simulink model "uavSafeLanding"  (R2023b)
settings: Solver=VariableStepAuto  StartTime=0.0  StopTime=inf  RelTol=1e-3
values from neighbouring files (symbols this model uses):
  DroneMass = 0.1    [controllerData.sldd]
  Dx = 1.5    [controllerData.sldd]
  Dy = 1.5    [controllerData.sldd]
  Dz = 2.5    [controllerData.sldd]
  Gravity = 9.81    [controllerData.sldd]
  Ix = 0.0    [controllerData.sldd]
  Iy = 0.0    [controllerData.sldd]
  Iz = 0.0    [controllerData.sldd]
  Nx = 10.0    [controllerData.sldd]
  Ny = 10.0    [controllerData.sldd]
  Nz = 14.4947065605712    [controllerData.sldd]
  Px = 6.0    [controllerData.sldd]
  Py = 6.0    [controllerData.sldd]
  Pz = 6.5    [controllerData.sldd]
undefined symbols (not defined in the file or in its folder): mission, rigidtform3d
libraries: slpidlib x6, uavalgslib x3, robotcorelib x2, simulink x1, sim3dphyssensorlib x1, sim3dlib x1, uavsim3dlib x1, uavutilslib x1
settings Model: DataDictionary=controllerData.sldd  Creator=The MathWorks, Inc.  LastModifiedBy=The MathWorks, Inc.
settings DebuggingCC: ParameterPrecisionLossMsg=none

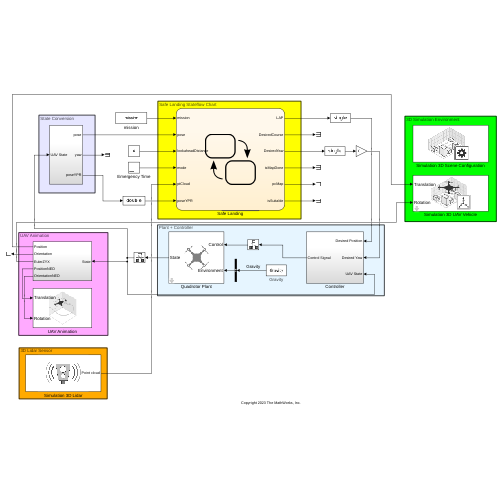
[thumbnail: Simulink's stored preview of the top-level diagram]
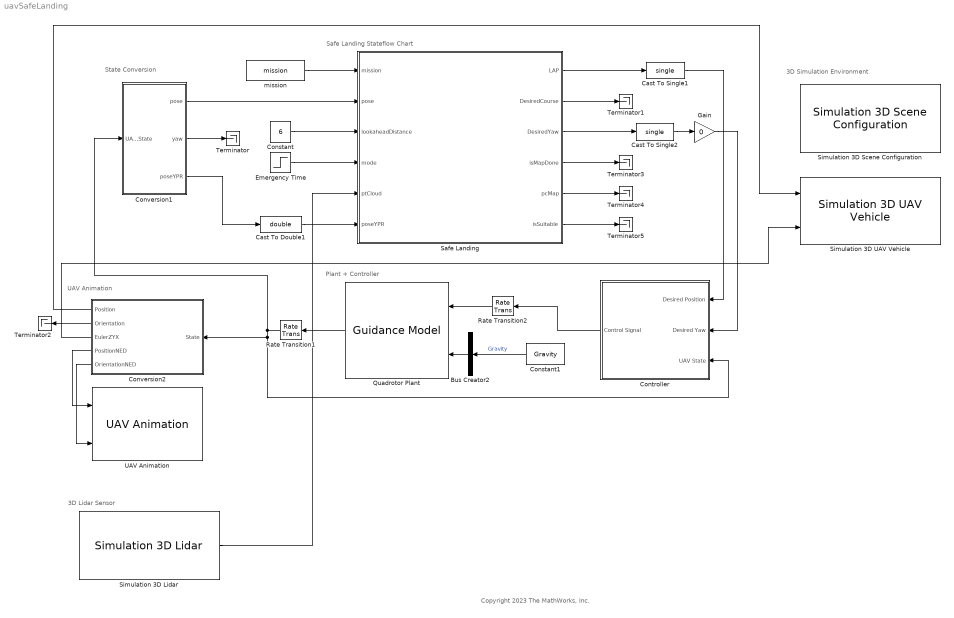
== system uavSafeLanding ==
  note: UAV Animation
  note: 3D Lidar Sensor
  note: Plant + Controller
  note: State Conversion
  note: 3D Simulation Environment
  note: Safe Landing Stateflow Chart
  note: Copyright 2023 The MathWorks, Inc.
  Bus Creator2 : BusCreator  Inputs=1  OutDataTypeStr=Bus: uavGuidanceEnvironmentBus  NonVirtualBus=on
  Cast To Double1 : DataTypeConversion  OutDataTypeStr=double  SaturateOnIntegerOverflow=off  RndMeth=Floor
  Cast To Single1 : DataTypeConversion  OutDataTypeStr=single  SaturateOnIntegerOverflow=off  RndMeth=Floor
  Cast To Single2 : DataTypeConversion  OutDataTypeStr=single  SaturateOnIntegerOverflow=off  RndMeth=Floor
  Constant : Constant  Value=6
  Constant1 : Constant  Value=Gravity  OutDataTypeStr=single
      settings: AttributesFormatString=%<Value>
  Controller : Subsystem
  Conversion1 : Subsystem
  Conversion2 : Subsystem
  Emergency Time : Step  Time=Time  Before=1  After=2  SampleTime=0  mask{Time=10}
      mask prompts: Time "Emergency time (s):"
      mask TypeOptions Time: Time
  Gain : Gain  Gain=0
  Quadrotor Plant : uavalgslib/Guidance Model  ModelType=MultirotorGuidance  SpecifiedDataType=single  SimulateUsing=Code generation  InitialWorldPositionMultirotor=[mission(1,1);mission(1,2);mission(1,3)]  InitialWorldVelocityMultirotor=[0; 0; 0]  InitialEulerZYXMultirotor=|  InitialBodyAngularRateRPYMultirotor=[0; 0; 0]  InitialThrustMultirotor=0  InitialNorthFixedWing=0  InitialEastFixedWing=0  InitialHeightFixedWing=0  InitialAirSpeedFixedWing=0  InitialHeadingAngleFixedWing=0  InitialFlightPathAngleFixedWing=0  InitialRollAngleFixedWing=0  InitialRollAngleRateFixedWing=0  PDRollMultirotor=[3402.97,116.67]  PDPitchMultirotor=[3402.97, 116.67]  PYawRateMultirotor=1950  PThrustMultirotor=3900  MassMultirotor=0.1  PHeightFixedWing=3.9  PHeadingAngleFixedWing=3.9  PFlightPathAngleFixedWing=39  PDRollFixedWing=[3402.97, 116.67]  PAirSpeedFixedWing=1  FlightPathAngleLimitsFixedWing=[-pi/2, pi/2]  StateBusName='uavGuidanceStateBus'  ControlBusName='uavGuidanceControlBus'  EnvironmentBusName='uavGuidanceEnvironmentBus'  DataType=single
      | [ 0
      | ;0;0]
  Rate Transition1 : RateTransition  OutPortSampleTime=UAVSampleTime
  Rate Transition2 : RateTransition  OutPortSampleTime=UAVSampleTime
  Safe Landing : Stateflow chart  TreatAsAtomicUnit=on  SystemSampleTime=0.1
  Simulation 3D Lidar : sim3dphyssensorlib/Simulation 3D Lidar  Priority=1  sensorTag=Sim3dSensor1  sensorId=1  sensorName=Sim3dSensor1  vehTagList={'Scene Origin';'SimulinkVehicle1'}  vehTag=SimulinkVehicle1  mountLoc=Origin  offsetFlag=on  tmountOffset=[0, 0, -1]  rmountOffset=[0, 90, 0]  DetectionRange=100  RangeResolution=0.03  VerticalFOV=30  VerticalResolution=2  HorizontalFOV=360  HorizontalResolution=0.2  DistanceOutportEnabled=off  ReflectivityOutportEnabled=off  SemanticOutportEnabled=off  TransformOutportEnabled=off  SampleTime=0.1  mountPoint=[0 0 -1]  mountOrientation=[0 -90 0]  aMode=4  ID=1
      settings: LibrarySourceBlock=uavsim3dlib/Simulation 3D Lidar
  Simulation 3D Scene Configuration : sim3dlib/Simulation 3D Scene Configuration  Priority=0  ProjectFormat=Default Scenes  SceneDesc=US city block  ProjectName=/mathworks/devel/bat/Bdoc23b/build/matlab/toolbox/shared/sim3d_projects/automotive_project_linux/UE/LinuxNoEditor/AutoVrtlEnv.sh  ScenePath=/Game/Maps/USCityBlock  EnableOpenDRIVE=off  vehTagList={'Custom';'Scene Origin';'SimulinkVehicle1'}  vehTag=SimulinkVehicle1  FreeCameraInitialTranslation=[0, 0, 0]  FreeCameraDefaultInitialTranslation=[-6, 0, 2]  FreeCameraInitialRotation=[0, 0, 0]  FreeCameraDefaultInitialRotation=[0, -15, 0]  OpVisEn=off  Ts=0.1  EnableWindow=on  EnableRemoteAccess=off  EnableWeather=off  SunAltitude=-57.600  SunAzimuth=90  clouds=67.0  wind=1  fog=98.0  rain=88.0  EnableGeospatial=off  OriginHeight=200  OriginLatitude=40.744652  OriginLongitude=-73.988864  MapStyle=Aerial  AdditionalAssetIDs=[]  UseAdvancedSunSky=off  SolarTime=11  TimeZone=-5  Day=21  Month=9  Year=2022  UseDaylightSavingTime=on  DSTStartDay=10  DSTStartMonth=3  DSTEndDay=3  DSTEndMonth=11  DSTSwitchHour=2  sensorTag=MainCamera1  sensorId=1  sensorName=MainCamera1  mountLoc=Origin  offsetFlag=off  tmountOffset=[0, 0, 0]  rmountOffset=[0, 0, 0]  HorizontalResolution=1280  VerticalResolution=720  HorizontalFOV=60  mountPoint=[0 0 0]  mountOrientation=[0 0 0]  aMode=4  ID=1  GeoTrigger=Inactive
      settings: LibrarySourceBlock=uavsim3dlib/Simulation 3D Scene Configuration
  Simulation 3D UAV Vehicle : uavsim3dlib/Simulation 3D UAV Vehicle  Priority=-1  Mesh=Quadrotor  MeshPath=/MathWorksUAVContent/UAVs/HexaRotorUAV/HexaRotor.HexaRotor  Color=Yellow  ActorName=SimulinkVehicle1  UseGlobalFrame=off  InitialTranslation=[mission(1,1) mission(1,2) mission(1,3)]  InitialRotation=[0 0 0]  InitialTranslationGlobal=[0 0 0]  InitialGeoOrigin=[0 0 0]  InitialRotationGlobal=[0 0 0]  SampleTime=-1  ActorType=SimulinkVehicle  ID=1  aMode=4  ActorTag=SimulinkVehicle1
  Terminator{,1..5} (6 alike) : Terminator
  UAV Animation : uavutilslib/UAV Animation  UAVType=Multirotor  UAVSize=1  InertialZDirection=Down  SampleTime=0.2
  mission : Constant  Value=mission
  wires:
  Emergency Time/1 -> Safe Landing/4(mode)
  Conversion1/2(yaw) -> Terminator/1
  Constant1/1 -> Bus Creator2/1  "Gravity"
  Cast To Single2/1 -> Gain/1
  Rate Transition2/1 -> Quadrotor Plant/1
  Conversion2/1(Position) -> Simulation 3D UAV Vehicle/1
  Safe Landing/3(DesiredYaw) -> Cast To Single2/1
  Cast To Single1/1 -> Controller/1(Desired Position)
  Conversion1/1(pose) -> Safe Landing/2(pose)
  Safe Landing/2(DesiredCourse) -> Terminator1/1
  Bus Creator2/1 -> Quadrotor Plant/2
  Rate Transition1/1 -> Controller/3(UAV State), Conversion2/1(State), Conversion1/1(UAV State)
  Gain/1 -> Controller/2(Desired Yaw)
  Constant/1 -> Safe Landing/3(lookaheadDistance)
  mission/1 -> Safe Landing/1(mission)
  Quadrotor Plant/1 -> Rate Transition1/1
  Controller/1(Control Signal) -> Rate Transition2/1
  Safe Landing/1(LAP) -> Cast To Single1/1
  Conversion1/3(poseYPR) -> Cast To Double1/1
  Cast To Double1/1 -> Safe Landing/6(poseYPR)
  Simulation 3D Lidar/1 -> Safe Landing/5(ptCloud)
  Conversion2/3(EulerZYX) -> Simulation 3D UAV Vehicle/2
  Conversion2/2(Orientation) -> Terminator2/1
  Safe Landing/4(isMapDone) -> Terminator3/1
  Safe Landing/5(pcMap) -> Terminator4/1
  Safe Landing/6(isSuitable) -> Terminator5/1
  Conversion2/4(PositionNED) -> UAV Animation/1
  Conversion2/5(OrientationNED) -> UAV Animation/2

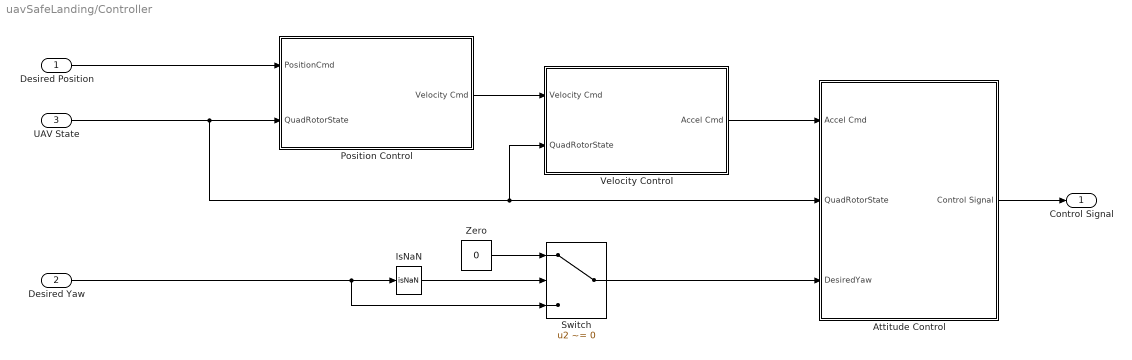
== system uavSafeLanding/Controller ==
  Desired Position : Inport
  Desired Yaw : Inport  Port=2
  UAV State : Inport  Port=3
  Attitude Control : Subsystem
  IsNaN : RelationalOperator  Operator=isNaN  OutDataTypeStr=boolean  RndMeth=Simplest  InputSameDT=off
  Position Control : Subsystem
  Switch : Switch  Criteria=u2 ~= 0  SaturateOnIntegerOverflow=off  InputSameDT=off
  Velocity Control : Subsystem
  Zero : Constant  Value=0  OutDataTypeStr=Inherit: Inherit via back propagation
  Control Signal : Outport
  wires:
  Desired Position/1 -> Position Control/1(PositionCmd)
  Velocity Control/1(Accel Cmd) -> Attitude Control/1(Accel Cmd)
  Attitude Control/1(Control Signal) -> Control Signal/1
  UAV State/1 -> Position Control/2(QuadRotorState), Velocity Control/2(QuadRotorState), Attitude Control/2(QuadRotorState)
  Position Control/1(Velocity Cmd) -> Velocity Control/1(Velocity Cmd)
  Zero/1 -> Switch/1
  IsNaN/1 -> Switch/2
  Desired Yaw/1 -> Switch/3, IsNaN/1
  Switch/1 -> Attitude Control/3(DesiredYaw)

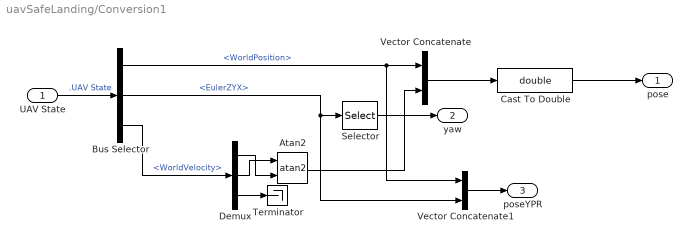
== system uavSafeLanding/Conversion1 ==
  UAV State : Inport
  Atan2 : Trigonometry  Operator=atan2
  Bus Selector : BusSelector  OutputSignals=WorldPosition,EulerZYX,WorldVelocity
  Cast To Double : DataTypeConversion  OutDataTypeStr=double  SaturateOnIntegerOverflow=off  RndMeth=Floor
  Demux : Demux  Outputs=3
  Selector : Selector  InputPortWidth=3  IndexOptions=Index vector (dialog)  Indices=[1]  OutputSizes=1
  Terminator : Terminator
  Vector Concatenate : Concatenate
  Vector Concatenate1 : Concatenate
  pose : Outport
  yaw : Outport  Port=2
  poseYPR : Outport  Port=3
  wires:
  Bus Selector/2 -> Vector Concatenate1/2, Selector/1  "<EulerZYX>"
  Bus Selector/1 -> Vector Concatenate1/1, Vector Concatenate/1  "<WorldPosition>"
  UAV State/1 -> Bus Selector/1  ".UAV State"
  Vector Concatenate/1 -> Cast To Double/1
  Bus Selector/3 -> Demux/1  "<WorldVelocity>"
  Demux/3 -> Terminator/1
  Atan2/1 -> Vector Concatenate/2
  Selector/1 -> yaw/1
  Demux/2 -> Atan2/1
  Demux/1 -> Atan2/2
  Vector Concatenate1/1 -> poseYPR/1
  Cast To Double/1 -> pose/1

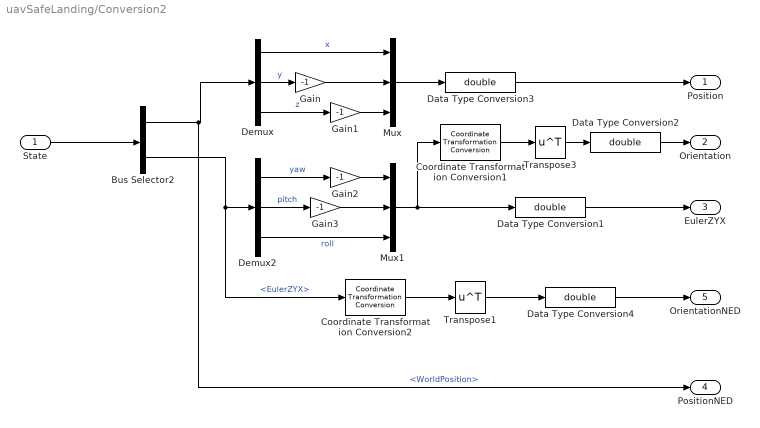
== system uavSafeLanding/Conversion2 ==
  State : Inport
  Bus Selector2 : BusSelector  OutputSignals=WorldPosition,EulerZYX
  Coordinate Transformation Conversion1 : robotcorelib/Coordinate Transformation Conversion  InputRepresentation=Euler Angles  InputEulerSequence=ZYX  ShowTrVecInputPort=on  OutputRepresentation=Quaternion  OutputEulerSequence=ZYX  ShowTrVecOutputPort=on  SimulateUsing=Code generation
  Coordinate Transformation Conversion2 : robotcorelib/Coordinate Transformation Conversion  InputRepresentation=Euler Angles  InputEulerSequence=ZYX  ShowTrVecInputPort=on  OutputRepresentation=Quaternion  OutputEulerSequence=ZYX  ShowTrVecOutputPort=on  SimulateUsing=Code generation
  Data Type Conversion{1..4} (4 alike) : DataTypeConversion  OutDataTypeStr=double  SaturateOnIntegerOverflow=off  RndMeth=Floor
  Demux : Demux  Outputs=3
  Demux2 : Demux  Outputs=3
  Gain{,1..3} (4 alike) : Gain  Gain=-1
  Mux : Mux  Inputs=3
  Mux1 : Mux  Inputs=3
  Transpose1 : Math  Operator=transpose
  Transpose3 : Math  Operator=transpose
  Position : Outport
  Orientation : Outport  Port=2
  EulerZYX : Outport  Port=3
  PositionNED : Outport  Port=4
  OrientationNED : Outport  Port=5
  wires:
  Bus Selector2/1 -> PositionNED/1, Demux/1  "<WorldPosition>"
  Gain3/1 -> Mux1/2
  Demux2/3 -> Mux1/3  "roll"
  State/1 -> Bus Selector2/1
  Demux/2 -> Gain/1  "y"
  Gain1/1 -> Mux/3
  Gain/1 -> Mux/2
  Demux/1 -> Mux/1  "x"
  Gain2/1 -> Mux1/1
  Demux2/1 -> Gain2/1  "yaw"
  Demux/3 -> Gain1/1  "z"
  Demux2/2 -> Gain3/1  "pitch"
  Mux/1 -> Data Type Conversion3/1
  Coordinate Transformation Conversion1/1 -> Transpose3/1
  Bus Selector2/2 -> Coordinate Transformation Conversion2/1, Demux2/1  "<EulerZYX>"
  Transpose3/1 -> Data Type Conversion2/1
  Mux1/1 -> Coordinate Transformation Conversion1/1, Data Type Conversion1/1
  Data Type Conversion3/1 -> Position/1
  Data Type Conversion2/1 -> Orientation/1
  Data Type Conversion1/1 -> EulerZYX/1
  Coordinate Transformation Conversion2/1 -> Transpose1/1
  Transpose1/1 -> Data Type Conversion4/1
  Data Type Conversion4/1 -> OrientationNED/1

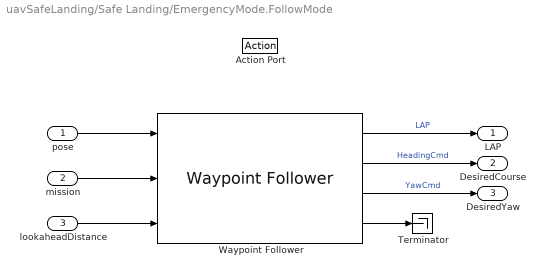
== system uavSafeLanding/Safe Landing/EmergencyMode.FollowMode ==
  pose : Inport
  mission : Inport  Port=2
  lookaheadDistance : Inport  Port=3
  Action Port : ActionPort
      settings: CopyFcn=Stateflow.SLINSF.SimulinkMan.removeBlockPreDeleteFcn  PreDeleteFcn=Stateflow.SLINSF.SimulinkMan.unsafePredeleteFcn
  Terminator : Terminator
  Waypoint Follower : uavalgslib/Waypoint Follower  UAVType=multirotor  StartFrom=closest  TransitionRadiusSource=internal  TransitionRadius=5  MinLookaheadDistance=0.1  YawInput=off  ShowCrossTrackErrorOutput=off  ShowStatusOutput=off  SimulateUsing=Interpreted execution
  LAP : Outport
  DesiredCourse : Outport  Port=2
  DesiredYaw : Outport  Port=3
  wires:
  mission/1 -> Waypoint Follower/2
  lookaheadDistance/1 -> Waypoint Follower/3
  Waypoint Follower/1 -> LAP/1  "LAP"
  pose/1 -> Waypoint Follower/1
  Waypoint Follower/4 -> Terminator/1
  Waypoint Follower/3 -> DesiredYaw/1  "YawCmd"
  Waypoint Follower/2 -> DesiredCourse/1  "HeadingCmd"

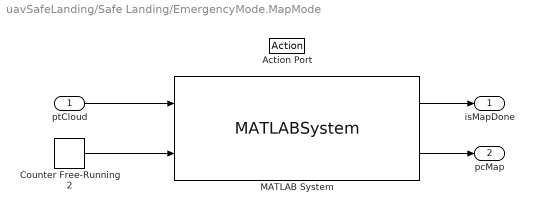
== system uavSafeLanding/Safe Landing/EmergencyMode.MapMode ==
  ptCloud : Inport
  Action Port : ActionPort
      settings: CopyFcn=Stateflow.SLINSF.SimulinkMan.removeBlockPreDeleteFcn  PreDeleteFcn=Stateflow.SLINSF.SimulinkMan.unsafePredeleteFcn
  Counter Free-Running2 : simulink/Sources/Counter Free-Running  NumBits=16  tsamp=-1
  MATLAB System : MATLABSystem  System=exampleHelperMapBuilder  mapGridSize=0.2  downsamplePercent=0.1  quadCopterROI=[ -2, 2, -2, 2, -2, 2 ]  sensorPoseWRTUAV=rigidtform3d( [ 90, 90, 0 ], [ 0, 0, 0 ] )  SimulateUsing=Interpreted execution
      mask Type: exampleHelperMapBuilder
      mask Display:
      | disp('exampleHelperMapBuilder');
      | port_label('input',1,'ptcloud');
      | port_label('input',2,'count');
      | port_label('output',1,'isMapDone');
      | port_label('output',2,'pcMap');
  isMapDone : Outport  OutDataTypeStr=boolean  PortDimensions=[1 1]
      settings: VarSizeSig=Yes
  pcMap : Outport  Port=2  OutDataTypeStr=double  PortDimensions=[600000 3]
  wires:
  ptCloud/1 -> MATLAB System/1
  Counter Free-Running2/1 -> MATLAB System/2
  MATLAB System/1 -> isMapDone/1
  MATLAB System/2 -> pcMap/1

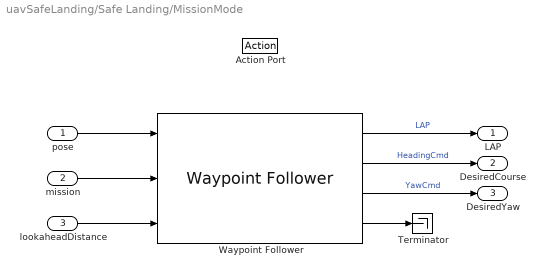
== system uavSafeLanding/Safe Landing/MissionMode ==
  pose : Inport
  mission : Inport  Port=2
  lookaheadDistance : Inport  Port=3
  Action Port : ActionPort
      settings: CopyFcn=Stateflow.SLINSF.SimulinkMan.removeBlockPreDeleteFcn  PreDeleteFcn=Stateflow.SLINSF.SimulinkMan.unsafePredeleteFcn
  Terminator : Terminator
  Waypoint Follower : uavalgslib/Waypoint Follower  UAVType=multirotor  StartFrom=first  TransitionRadiusSource=internal  TransitionRadius=5  MinLookaheadDistance=0.1  YawInput=off  ShowCrossTrackErrorOutput=off  ShowStatusOutput=off  SimulateUsing=Interpreted execution
  LAP : Outport
  DesiredCourse : Outport  Port=2
  DesiredYaw : Outport  Port=3
  wires:
  mission/1 -> Waypoint Follower/2
  lookaheadDistance/1 -> Waypoint Follower/3
  Waypoint Follower/1 -> LAP/1  "LAP"
  pose/1 -> Waypoint Follower/1
  Waypoint Follower/4 -> Terminator/1
  Waypoint Follower/3 -> DesiredYaw/1  "YawCmd"
  Waypoint Follower/2 -> DesiredCourse/1  "HeadingCmd"

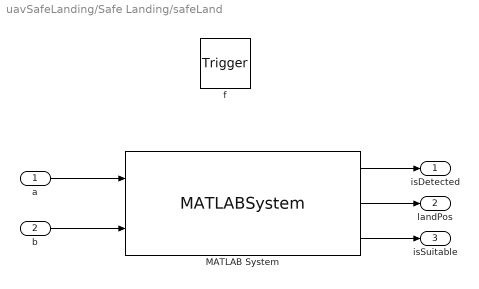
== system uavSafeLanding/Safe Landing/safeLand ==
  a : Inport  OutDataTypeStr=double  PortDimensions=[600000 3]
  b : Inport  Port=2  OutDataTypeStr=double  PortDimensions=[3 1]
  f : TriggerPort  TriggerType=function-call  VariantControl=(inherit)
      settings: CopyFcn=Stateflow.SLINSF.SimulinkMan.removeBlockPreDeleteFcn  PreDeleteFcn=Stateflow.SLINSF.SimulinkMan.unsafePredeleteFcn
  MATLAB System : MATLABSystem  System=exampleHelperSafeLanding  innerBlockSize=[ 20, 20 ]  radius=5  gridSize=3  minPoints=10  verticalVarianceThreshold=0.5  slopeThreshold=6  residualThreshold=10  reliefThreshold=3  weight=[ 1, 1, 1, 1 ]  qualityThreshold=1  pcDownsamplePercent=0.1  SimulateUsing=Interpreted execution
      mask Type: exampleHelperSafeLanding
      mask Display:
      | disp('exampleHelperSafeLanding');
      | port_label('input',1,'ptCloudMap');
      | port_label('input',2,'uavStartPosition');
      | port_label('output',1,'isDetected');
      | port_label('output',2,'bestLandingZone');
      | port_label('output',3,'isSuitable');
  isDetected : Outport
  landPos : Outport  Port=2
  isSuitable : Outport  Port=3
  wires:
  a/1 -> MATLAB System/1
  b/1 -> MATLAB System/2
  MATLAB System/1 -> isDetected/1
  MATLAB System/2 -> landPos/1
  MATLAB System/3 -> isSuitable/1

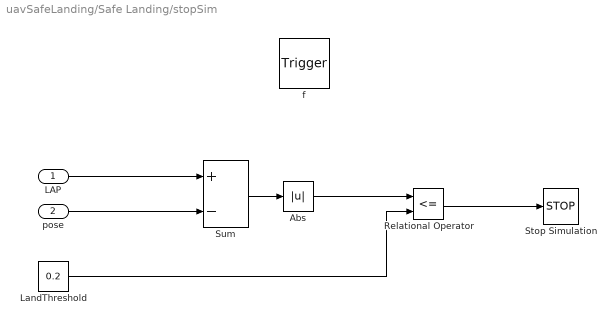
== system uavSafeLanding/Safe Landing/stopSim ==
  LAP : Inport  OutDataTypeStr=double  PortDimensions=1
  pose : Inport  Port=2  OutDataTypeStr=double  PortDimensions=1
  f : TriggerPort  TriggerType=function-call  VariantControl=(inherit)
      settings: CopyFcn=Stateflow.SLINSF.SimulinkMan.removeBlockPreDeleteFcn  PreDeleteFcn=Stateflow.SLINSF.SimulinkMan.unsafePredeleteFcn
  Abs : Abs  SaturateOnIntegerOverflow=off
  LandThreshold : Constant  Value=0.2
  Relational Operator : RelationalOperator  Operator=<=  OutDataTypeStr=boolean  RndMeth=Simplest  InputSameDT=off
  Stop Simulation : Stop
  Sum : Sum  Inputs=+-
  wires:
  LandThreshold/1 -> Relational Operator/2
  Relational Operator/1 -> Stop Simulation/1
  LAP/1 -> Sum/1
  Sum/1 -> Abs/1
  Abs/1 -> Relational Operator/1
  pose/1 -> Sum/2

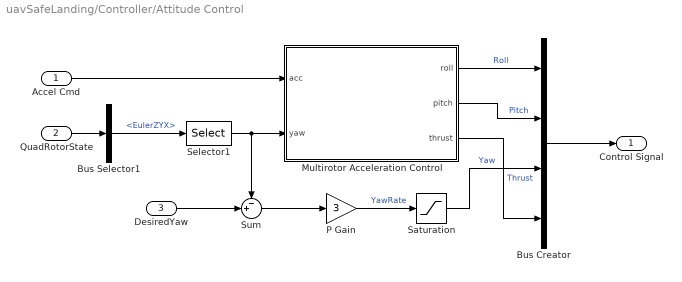
== system uavSafeLanding/Controller/Attitude Control ==
  Accel Cmd : Inport
  QuadRotorState : Inport  Port=2
  DesiredYaw : Inport  Port=3
  Bus Creator : BusCreator  Inputs=4  OutDataTypeStr=Bus: uavGuidanceControlBus  NonVirtualBus=on
      settings: InheritFromInputs=off
  Bus Selector1 : BusSelector  OutputSignals=EulerZYX
  Multirotor Acceleration Control : MATLAB Function  TreatAsAtomicUnit=on
  P Gain : Gain  Gain=3
  Saturation : Saturate
  Selector1 : Selector  InputPortWidth=3  IndexOptions=Index vector (dialog)  Indices=[1]  OutputSizes=1
  Sum : Sum  Inputs=-+|
  Control Signal : Outport
  wires:
  Selector1/1 -> Multirotor Acceleration Control/2(yaw), Sum/1
  Bus Creator/1 -> Control Signal/1
  Sum/1 -> P Gain/1
  Multirotor Acceleration Control/1(roll) -> Bus Creator/1  "Roll"
  Multirotor Acceleration Control/2(pitch) -> Bus Creator/2  "Pitch"
  Multirotor Acceleration Control/3(thrust) -> Bus Creator/4  "Thrust"
  P Gain/1 -> Saturation/1  "YawRate"
  Accel Cmd/1 -> Multirotor Acceleration Control/1(acc)
  QuadRotorState/1 -> Bus Selector1/1
  Bus Selector1/1 -> Selector1/1  "<EulerZYX>"
  Saturation/1 -> Bus Creator/3  "Yaw"
  DesiredYaw/1 -> Sum/2

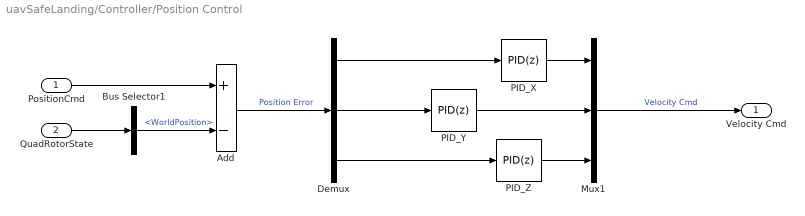
== system uavSafeLanding/Controller/Position Control ==
  PositionCmd : Inport
  QuadRotorState : Inport  Port=2
  Add : Sum  Inputs=+-
  Bus Selector1 : BusSelector  OutputSignals=WorldPosition
  Demux : Demux  Outputs=3
  Mux1 : Mux  Inputs=3
  PID_X : slpidlib/PID Controller  Controller=PID  Form=Parallel  TimeDomain=Discrete-time  UseExternalTs=off  SampleTime=-1  IntegratorMethod=Forward Euler  FilterMethod=Forward Euler  ControllerParametersSource=internal  P=Px  I=Ix  UseKiTs=off  D=Dx  N=Nx  UseFilter=on  TunerSelectOption=Transfer Function Based (PID Tuner App)  InitialConditionSource=internal  InitialConditionForIntegrator=0  InitialConditionForFilter=0  DifferentiatorICPrevScaledInput=0  ExternalReset=none  TrackingMode=off  Kt=1  LimitOutput=on  SatLimitsSource=internal  UpperSaturationLimit=3  LowerSaturationLimit=-3  LinearizeAsGain=on  AntiWindupMode=clamping  Kb=1  LimitIntegrator=off  UpperIntegratorSaturationLimit=inf  LowerIntegratorSaturationLimit=-inf  POutMin=[]  POutMax=[]  IOutMin=[]  IOutMax=[]  DOutMin=[]  DOutMax=[]  NOutMin=[]  NOutMax=[]  SumOutMin=[]  SumOutMax=[]  SaturationOutMin=[]  SaturationOutMax=[]  PParamMin=[]  PParamMax=[]  IParamMin=[]  IParamMax=[]  DParamMin=[]  DParamMax=[]  NParamMin=[]  NParamMax=[]  KbParamMin=[]  KbParamMax=[]  KtParamMin=[]  KtParamMax=[]  KbOutMin=[]  KbOutMax=[]  KtOutMin=[]  KtOutMax=[]  IntegratorOutMin=[]  IntegratorOutMax=[]  FilterOutMin=[]  FilterOutMax=[]  SumI1OutMin=SumI1OutMin  SumI1OutMax=SumI1OutMax  SumI2OutMin=[]  SumI2OutMax=[]  SumI3OutMin=[]  SumI3OutMax=[]  SumI4OutMin=[]  SumI4OutMax=[]  SumDOutMin=[]  SumDOutMax=[]  DifferentiatorOutMin=[]  DifferentiatorOutMax=[]  FilterDiffOutCoefMin=[]  FilterDiffOutCoefMax=[]  ReciprocalOutMin=[]  ReciprocalOutMax=[]  SumDenOutMin=[]  SumDenOutMax=[]  SumNumOutMin=[]  SumNumOutMax=[]  DivideOutMin=[]  DivideOutMax=[]  UdiffTsProdOutMin=[]  UdiffTsProdOutMax=[]  NTsProdOutMin=[]  NTsProdOutMax=[]  UintegralTsProdOutMin=[]  UintegralTsProdOutMax=[]  UngainTsProdOutMin=[]  UngainTsProdOutMax=[]  ClampingZeroOutDataTypeStr=Inherit: Inherit via back propagation  ClampingZeroOutMin=[]  ClampingZeroOutMax=[]  FilterDenConstantOutDataTypeStr=Inherit: Inherit via back propagation  FilterDenConstantOutMin=[]  FilterDenConstantOutMax=[]  PCopyOutDataTypeStr=Inherit: Inherit via back propagation  PCopyOutMin=[]  PCopyOutMax=[]  NCopyOutDataTypeStr=Inherit: Inherit via back propagation  NCopyOutMin=[]  NCopyOutMax=[]  IntegratorContinuousStateAttributes=''  IntegratorStateMustResolveToSignalObject=off  IntegratorRTWStateStorageClass=Auto  FilterContinuousStateAttributes=''  FilterStateMustResolveToSignalObject=off  FilterRTWStateStorageClass=Auto  ParallelPVariant=InternalParameters  IdealPVariant=Disabled  IVariant=InternalParameters  DVariant=InternalParameters  IntegratorVariant=Discrete  SatVariant=Enabled  AWVariant=DiscClampingParallel  PCopyVariant=Disabled  TRVariant=Disabled  FdbkBlocksVariant=Forward  IdealPFdbkVariant=Disabled  SatFdbkVariant=Disabled  DerivativeFilterVariant=ForwardEulerFilter  NVariant=InternalParameters  NCopyVariant=Disabled  FilterICVariant=InternalICsFilter  IntegratorICVariant=InternalICs  ExternalResetVariant=Disabled  TRSumVariant=Passthrough  SumFdbkVariant=Disabled  SumVariant=Sum_PID  TsampFilterVariant=InternalTs  TsampNgainVariant=Passthrough  TsampIntegralVariant=Disabled_SignalSpec  ExternalSaturationOutDataTypeStr=Inherit: Same as second input
      settings: AttributesFormatString=P: %<P>, I: %<I>, D:%<D>
  PID_Y : slpidlib/PID Controller  Controller=PID  Form=Parallel  TimeDomain=Discrete-time  UseExternalTs=off  SampleTime=-1  IntegratorMethod=Forward Euler  FilterMethod=Forward Euler  ControllerParametersSource=internal  P=Py  I=Iy  UseKiTs=off  D=Dy  N=Ny  UseFilter=on  TunerSelectOption=Transfer Function Based (PID Tuner App)  InitialConditionSource=internal  InitialConditionForIntegrator=0  InitialConditionForFilter=0  DifferentiatorICPrevScaledInput=0  ExternalReset=none  TrackingMode=off  Kt=1  LimitOutput=on  SatLimitsSource=internal  UpperSaturationLimit=3  LowerSaturationLimit=-3  LinearizeAsGain=on  AntiWindupMode=clamping  Kb=1  LimitIntegrator=off  UpperIntegratorSaturationLimit=inf  LowerIntegratorSaturationLimit=-inf  POutMin=[]  POutMax=[]  IOutMin=[]  IOutMax=[]  DOutMin=[]  DOutMax=[]  NOutMin=[]  NOutMax=[]  SumOutMin=[]  SumOutMax=[]  SaturationOutMin=[]  SaturationOutMax=[]  PParamMin=[]  PParamMax=[]  IParamMin=[]  IParamMax=[]  DParamMin=[]  DParamMax=[]  NParamMin=[]  NParamMax=[]  KbParamMin=[]  KbParamMax=[]  KtParamMin=[]  KtParamMax=[]  KbOutMin=[]  KbOutMax=[]  KtOutMin=[]  KtOutMax=[]  IntegratorOutMin=[]  IntegratorOutMax=[]  FilterOutMin=[]  FilterOutMax=[]  SumI1OutMin=SumI1OutMin  SumI1OutMax=SumI1OutMax  SumI2OutMin=[]  SumI2OutMax=[]  SumI3OutMin=[]  SumI3OutMax=[]  SumI4OutMin=[]  SumI4OutMax=[]  SumDOutMin=[]  SumDOutMax=[]  DifferentiatorOutMin=[]  DifferentiatorOutMax=[]  FilterDiffOutCoefMin=[]  FilterDiffOutCoefMax=[]  ReciprocalOutMin=[]  ReciprocalOutMax=[]  SumDenOutMin=[]  SumDenOutMax=[]  SumNumOutMin=[]  SumNumOutMax=[]  DivideOutMin=[]  DivideOutMax=[]  UdiffTsProdOutMin=[]  UdiffTsProdOutMax=[]  NTsProdOutMin=[]  NTsProdOutMax=[]  UintegralTsProdOutMin=[]  UintegralTsProdOutMax=[]  UngainTsProdOutMin=[]  UngainTsProdOutMax=[]  ClampingZeroOutDataTypeStr=Inherit: Inherit via back propagation  ClampingZeroOutMin=[]  ClampingZeroOutMax=[]  FilterDenConstantOutDataTypeStr=Inherit: Inherit via back propagation  FilterDenConstantOutMin=[]  FilterDenConstantOutMax=[]  PCopyOutDataTypeStr=Inherit: Inherit via back propagation  PCopyOutMin=[]  PCopyOutMax=[]  NCopyOutDataTypeStr=Inherit: Inherit via back propagation  NCopyOutMin=[]  NCopyOutMax=[]  IntegratorContinuousStateAttributes=''  IntegratorStateMustResolveToSignalObject=off  IntegratorRTWStateStorageClass=Auto  FilterContinuousStateAttributes=''  FilterStateMustResolveToSignalObject=off  FilterRTWStateStorageClass=Auto  ParallelPVariant=InternalParameters  IdealPVariant=Disabled  IVariant=InternalParameters  DVariant=InternalParameters  IntegratorVariant=Discrete  SatVariant=Enabled  AWVariant=DiscClampingParallel  PCopyVariant=Disabled  TRVariant=Disabled  FdbkBlocksVariant=Forward  IdealPFdbkVariant=Disabled  SatFdbkVariant=Disabled  DerivativeFilterVariant=ForwardEulerFilter  NVariant=InternalParameters  NCopyVariant=Disabled  FilterICVariant=InternalICsFilter  IntegratorICVariant=InternalICs  ExternalResetVariant=Disabled  TRSumVariant=Passthrough  SumFdbkVariant=Disabled  SumVariant=Sum_PID  TsampFilterVariant=InternalTs  TsampNgainVariant=Passthrough  TsampIntegralVariant=Disabled_SignalSpec  ExternalSaturationOutDataTypeStr=Inherit: Same as second input
      settings: AttributesFormatString=P: %<P>, I: %<I>, D:%<D>
  PID_Z : slpidlib/PID Controller  Controller=PID  Form=Parallel  TimeDomain=Discrete-time  UseExternalTs=off  SampleTime=-1  IntegratorMethod=Forward Euler  FilterMethod=Forward Euler  ControllerParametersSource=internal  P=Pz  I=Iz  UseKiTs=off  D=Dz  N=Nz  UseFilter=on  TunerSelectOption=Transfer Function Based (PID Tuner App)  InitialConditionSource=internal  InitialConditionForIntegrator=0  InitialConditionForFilter=0  DifferentiatorICPrevScaledInput=0  ExternalReset=none  TrackingMode=off  Kt=1  LimitOutput=on  SatLimitsSource=internal  UpperSaturationLimit=3  LowerSaturationLimit=-3  LinearizeAsGain=on  AntiWindupMode=clamping  Kb=1  LimitIntegrator=off  UpperIntegratorSaturationLimit=inf  LowerIntegratorSaturationLimit=-inf  POutMin=[]  POutMax=[]  IOutMin=[]  IOutMax=[]  DOutMin=[]  DOutMax=[]  NOutMin=[]  NOutMax=[]  SumOutMin=[]  SumOutMax=[]  SaturationOutMin=[]  SaturationOutMax=[]  PParamMin=[]  PParamMax=[]  IParamMin=[]  IParamMax=[]  DParamMin=[]  DParamMax=[]  NParamMin=[]  NParamMax=[]  KbParamMin=[]  KbParamMax=[]  KtParamMin=[]  KtParamMax=[]  KbOutMin=[]  KbOutMax=[]  KtOutMin=[]  KtOutMax=[]  IntegratorOutMin=[]  IntegratorOutMax=[]  FilterOutMin=[]  FilterOutMax=[]  SumI1OutMin=SumI1OutMin  SumI1OutMax=SumI1OutMax  SumI2OutMin=[]  SumI2OutMax=[]  SumI3OutMin=[]  SumI3OutMax=[]  SumI4OutMin=[]  SumI4OutMax=[]  SumDOutMin=[]  SumDOutMax=[]  DifferentiatorOutMin=[]  DifferentiatorOutMax=[]  FilterDiffOutCoefMin=[]  FilterDiffOutCoefMax=[]  ReciprocalOutMin=[]  ReciprocalOutMax=[]  SumDenOutMin=[]  SumDenOutMax=[]  SumNumOutMin=[]  SumNumOutMax=[]  DivideOutMin=[]  DivideOutMax=[]  UdiffTsProdOutMin=[]  UdiffTsProdOutMax=[]  NTsProdOutMin=[]  NTsProdOutMax=[]  UintegralTsProdOutMin=[]  UintegralTsProdOutMax=[]  UngainTsProdOutMin=[]  UngainTsProdOutMax=[]  ClampingZeroOutDataTypeStr=Inherit: Inherit via back propagation  ClampingZeroOutMin=[]  ClampingZeroOutMax=[]  FilterDenConstantOutDataTypeStr=Inherit: Inherit via back propagation  FilterDenConstantOutMin=[]  FilterDenConstantOutMax=[]  PCopyOutDataTypeStr=Inherit: Inherit via back propagation  PCopyOutMin=[]  PCopyOutMax=[]  NCopyOutDataTypeStr=Inherit: Inherit via back propagation  NCopyOutMin=[]  NCopyOutMax=[]  IntegratorContinuousStateAttributes=''  IntegratorStateMustResolveToSignalObject=off  IntegratorRTWStateStorageClass=Auto  FilterContinuousStateAttributes=''  FilterStateMustResolveToSignalObject=off  FilterRTWStateStorageClass=Auto  ParallelPVariant=InternalParameters  IdealPVariant=Disabled  IVariant=InternalParameters  DVariant=InternalParameters  IntegratorVariant=Discrete  SatVariant=Enabled  AWVariant=DiscClampingParallel  PCopyVariant=Disabled  TRVariant=Disabled  FdbkBlocksVariant=Forward  IdealPFdbkVariant=Disabled  SatFdbkVariant=Disabled  DerivativeFilterVariant=ForwardEulerFilter  NVariant=InternalParameters  NCopyVariant=Disabled  FilterICVariant=InternalICsFilter  IntegratorICVariant=InternalICs  ExternalResetVariant=Disabled  TRSumVariant=Passthrough  SumFdbkVariant=Disabled  SumVariant=Sum_PID  TsampFilterVariant=InternalTs  TsampNgainVariant=Passthrough  TsampIntegralVariant=Disabled_SignalSpec  ExternalSaturationOutDataTypeStr=Inherit: Same as second input
      settings: AttributesFormatString=P: %<P>, I: %<I>, D:%<D>
  Velocity Cmd : Outport
  wires:
  Demux/3 -> PID_Z/1
  Demux/1 -> PID_X/1
  PID_Z/1 -> Mux1/3
  Add/1 -> Demux/1  "Position Error"
  Demux/2 -> PID_Y/1
  Mux1/1 -> Velocity Cmd/1  "Velocity Cmd"
  PID_X/1 -> Mux1/1
  PID_Y/1 -> Mux1/2
  Bus Selector1/1 -> Add/2  "<WorldPosition>"
  QuadRotorState/1 -> Bus Selector1/1
  PositionCmd/1 -> Add/1

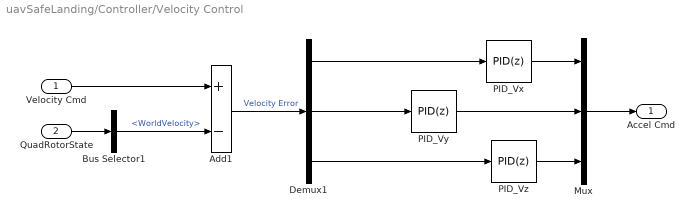
== system uavSafeLanding/Controller/Velocity Control ==
  Velocity Cmd : Inport
  QuadRotorState : Inport  Port=2
  Add1 : Sum  Inputs=+-
  Bus Selector1 : BusSelector  OutputSignals=WorldVelocity
  Demux1 : Demux  Outputs=3
  Mux : Mux  Inputs=3
  PID_Vx : slpidlib/PID Controller  Controller=PID  Form=Parallel  TimeDomain=Discrete-time  UseExternalTs=off  SampleTime=-1  IntegratorMethod=Forward Euler  FilterMethod=Forward Euler  ControllerParametersSource=internal  P=Px  I=Ix  UseKiTs=off  D=Dx  N=Nx  UseFilter=on  TunerSelectOption=Transfer Function Based (PID Tuner App)  InitialConditionSource=internal  InitialConditionForIntegrator=0  InitialConditionForFilter=0  DifferentiatorICPrevScaledInput=0  ExternalReset=none  TrackingMode=off  Kt=1  LimitOutput=on  SatLimitsSource=internal  UpperSaturationLimit=1  LowerSaturationLimit=-1  LinearizeAsGain=on  AntiWindupMode=clamping  Kb=1  LimitIntegrator=off  UpperIntegratorSaturationLimit=inf  LowerIntegratorSaturationLimit=-inf  POutMin=[]  POutMax=[]  IOutMin=[]  IOutMax=[]  DOutMin=[]  DOutMax=[]  NOutMin=[]  NOutMax=[]  SumOutMin=[]  SumOutMax=[]  SaturationOutMin=[]  SaturationOutMax=[]  PParamMin=[]  PParamMax=[]  IParamMin=[]  IParamMax=[]  DParamMin=[]  DParamMax=[]  NParamMin=[]  NParamMax=[]  KbParamMin=[]  KbParamMax=[]  KtParamMin=[]  KtParamMax=[]  KbOutMin=[]  KbOutMax=[]  KtOutMin=[]  KtOutMax=[]  IntegratorOutMin=[]  IntegratorOutMax=[]  FilterOutMin=[]  FilterOutMax=[]  SumI1OutMin=SumI1OutMin  SumI1OutMax=SumI1OutMax  SumI2OutMin=[]  SumI2OutMax=[]  SumI3OutMin=[]  SumI3OutMax=[]  SumI4OutMin=[]  SumI4OutMax=[]  SumDOutMin=[]  SumDOutMax=[]  DifferentiatorOutMin=[]  DifferentiatorOutMax=[]  FilterDiffOutCoefMin=[]  FilterDiffOutCoefMax=[]  ReciprocalOutMin=[]  ReciprocalOutMax=[]  SumDenOutMin=[]  SumDenOutMax=[]  SumNumOutMin=[]  SumNumOutMax=[]  DivideOutMin=[]  DivideOutMax=[]  UdiffTsProdOutMin=[]  UdiffTsProdOutMax=[]  NTsProdOutMin=[]  NTsProdOutMax=[]  UintegralTsProdOutMin=[]  UintegralTsProdOutMax=[]  UngainTsProdOutMin=[]  UngainTsProdOutMax=[]  ClampingZeroOutDataTypeStr=Inherit: Inherit via back propagation  ClampingZeroOutMin=[]  ClampingZeroOutMax=[]  FilterDenConstantOutDataTypeStr=Inherit: Inherit via back propagation  FilterDenConstantOutMin=[]  FilterDenConstantOutMax=[]  PCopyOutDataTypeStr=Inherit: Inherit via back propagation  PCopyOutMin=[]  PCopyOutMax=[]  NCopyOutDataTypeStr=Inherit: Inherit via back propagation  NCopyOutMin=[]  NCopyOutMax=[]  IntegratorContinuousStateAttributes=''  IntegratorStateMustResolveToSignalObject=off  IntegratorRTWStateStorageClass=Auto  FilterContinuousStateAttributes=''  FilterStateMustResolveToSignalObject=off  FilterRTWStateStorageClass=Auto  ParallelPVariant=InternalParameters  IdealPVariant=Disabled  IVariant=InternalParameters  DVariant=InternalParameters  IntegratorVariant=Discrete  SatVariant=Enabled  AWVariant=DiscClampingParallel  PCopyVariant=Disabled  TRVariant=Disabled  FdbkBlocksVariant=Forward  IdealPFdbkVariant=Disabled  SatFdbkVariant=Disabled  DerivativeFilterVariant=ForwardEulerFilter  NVariant=InternalParameters  NCopyVariant=Disabled  FilterICVariant=InternalICsFilter  IntegratorICVariant=InternalICs  ExternalResetVariant=Disabled  TRSumVariant=Passthrough  SumFdbkVariant=Disabled  SumVariant=Sum_PID  TsampFilterVariant=InternalTs  TsampNgainVariant=Passthrough  TsampIntegralVariant=Disabled_SignalSpec  ExternalSaturationOutDataTypeStr=Inherit: Same as second input
      settings: AttributesFormatString=P: %<P>, I: %<I>, D:%<D>
  PID_Vy : slpidlib/PID Controller  Controller=PID  Form=Parallel  TimeDomain=Discrete-time  UseExternalTs=off  SampleTime=-1  IntegratorMethod=Forward Euler  FilterMethod=Forward Euler  ControllerParametersSource=internal  P=Py  I=Iy  UseKiTs=off  D=Dy  N=Ny  UseFilter=on  TunerSelectOption=Transfer Function Based (PID Tuner App)  InitialConditionSource=internal  InitialConditionForIntegrator=0  InitialConditionForFilter=0  DifferentiatorICPrevScaledInput=0  ExternalReset=none  TrackingMode=off  Kt=1  LimitOutput=on  SatLimitsSource=internal  UpperSaturationLimit=1  LowerSaturationLimit=-1  LinearizeAsGain=on  AntiWindupMode=clamping  Kb=1  LimitIntegrator=off  UpperIntegratorSaturationLimit=inf  LowerIntegratorSaturationLimit=-inf  POutMin=[]  POutMax=[]  IOutMin=[]  IOutMax=[]  DOutMin=[]  DOutMax=[]  NOutMin=[]  NOutMax=[]  SumOutMin=[]  SumOutMax=[]  SaturationOutMin=[]  SaturationOutMax=[]  PParamMin=[]  PParamMax=[]  IParamMin=[]  IParamMax=[]  DParamMin=[]  DParamMax=[]  NParamMin=[]  NParamMax=[]  KbParamMin=[]  KbParamMax=[]  KtParamMin=[]  KtParamMax=[]  KbOutMin=[]  KbOutMax=[]  KtOutMin=[]  KtOutMax=[]  IntegratorOutMin=[]  IntegratorOutMax=[]  FilterOutMin=[]  FilterOutMax=[]  SumI1OutMin=SumI1OutMin  SumI1OutMax=SumI1OutMax  SumI2OutMin=[]  SumI2OutMax=[]  SumI3OutMin=[]  SumI3OutMax=[]  SumI4OutMin=[]  SumI4OutMax=[]  SumDOutMin=[]  SumDOutMax=[]  DifferentiatorOutMin=[]  DifferentiatorOutMax=[]  FilterDiffOutCoefMin=[]  FilterDiffOutCoefMax=[]  ReciprocalOutMin=[]  ReciprocalOutMax=[]  SumDenOutMin=[]  SumDenOutMax=[]  SumNumOutMin=[]  SumNumOutMax=[]  DivideOutMin=[]  DivideOutMax=[]  UdiffTsProdOutMin=[]  UdiffTsProdOutMax=[]  NTsProdOutMin=[]  NTsProdOutMax=[]  UintegralTsProdOutMin=[]  UintegralTsProdOutMax=[]  UngainTsProdOutMin=[]  UngainTsProdOutMax=[]  ClampingZeroOutDataTypeStr=Inherit: Inherit via back propagation  ClampingZeroOutMin=[]  ClampingZeroOutMax=[]  FilterDenConstantOutDataTypeStr=Inherit: Inherit via back propagation  FilterDenConstantOutMin=[]  FilterDenConstantOutMax=[]  PCopyOutDataTypeStr=Inherit: Inherit via back propagation  PCopyOutMin=[]  PCopyOutMax=[]  NCopyOutDataTypeStr=Inherit: Inherit via back propagation  NCopyOutMin=[]  NCopyOutMax=[]  IntegratorContinuousStateAttributes=''  IntegratorStateMustResolveToSignalObject=off  IntegratorRTWStateStorageClass=Auto  FilterContinuousStateAttributes=''  FilterStateMustResolveToSignalObject=off  FilterRTWStateStorageClass=Auto  ParallelPVariant=InternalParameters  IdealPVariant=Disabled  IVariant=InternalParameters  DVariant=InternalParameters  IntegratorVariant=Discrete  SatVariant=Enabled  AWVariant=DiscClampingParallel  PCopyVariant=Disabled  TRVariant=Disabled  FdbkBlocksVariant=Forward  IdealPFdbkVariant=Disabled  SatFdbkVariant=Disabled  DerivativeFilterVariant=ForwardEulerFilter  NVariant=InternalParameters  NCopyVariant=Disabled  FilterICVariant=InternalICsFilter  IntegratorICVariant=InternalICs  ExternalResetVariant=Disabled  TRSumVariant=Passthrough  SumFdbkVariant=Disabled  SumVariant=Sum_PID  TsampFilterVariant=InternalTs  TsampNgainVariant=Passthrough  TsampIntegralVariant=Disabled_SignalSpec  ExternalSaturationOutDataTypeStr=Inherit: Same as second input
      settings: AttributesFormatString=P: %<P>, I: %<I>, D:%<D>
  PID_Vz : slpidlib/PID Controller  Controller=PID  Form=Parallel  TimeDomain=Discrete-time  UseExternalTs=off  SampleTime=-1  IntegratorMethod=Forward Euler  FilterMethod=Forward Euler  ControllerParametersSource=internal  P=Pz  I=Iz  UseKiTs=off  D=Dz  N=Nz  UseFilter=on  TunerSelectOption=Transfer Function Based (PID Tuner App)  InitialConditionSource=internal  InitialConditionForIntegrator=0  InitialConditionForFilter=0  DifferentiatorICPrevScaledInput=0  ExternalReset=none  TrackingMode=off  Kt=1  LimitOutput=on  SatLimitsSource=internal  UpperSaturationLimit=4  LowerSaturationLimit=-4  LinearizeAsGain=on  AntiWindupMode=clamping  Kb=1  LimitIntegrator=off  UpperIntegratorSaturationLimit=inf  LowerIntegratorSaturationLimit=-inf  POutMin=[]  POutMax=[]  IOutMin=[]  IOutMax=[]  DOutMin=[]  DOutMax=[]  NOutMin=[]  NOutMax=[]  SumOutMin=[]  SumOutMax=[]  SaturationOutMin=[]  SaturationOutMax=[]  PParamMin=[]  PParamMax=[]  IParamMin=[]  IParamMax=[]  DParamMin=[]  DParamMax=[]  NParamMin=[]  NParamMax=[]  KbParamMin=[]  KbParamMax=[]  KtParamMin=[]  KtParamMax=[]  KbOutMin=[]  KbOutMax=[]  KtOutMin=[]  KtOutMax=[]  IntegratorOutMin=[]  IntegratorOutMax=[]  FilterOutMin=[]  FilterOutMax=[]  SumI1OutMin=SumI1OutMin  SumI1OutMax=SumI1OutMax  SumI2OutMin=[]  SumI2OutMax=[]  SumI3OutMin=[]  SumI3OutMax=[]  SumI4OutMin=[]  SumI4OutMax=[]  SumDOutMin=[]  SumDOutMax=[]  DifferentiatorOutMin=[]  DifferentiatorOutMax=[]  FilterDiffOutCoefMin=[]  FilterDiffOutCoefMax=[]  ReciprocalOutMin=[]  ReciprocalOutMax=[]  SumDenOutMin=[]  SumDenOutMax=[]  SumNumOutMin=[]  SumNumOutMax=[]  DivideOutMin=[]  DivideOutMax=[]  UdiffTsProdOutMin=[]  UdiffTsProdOutMax=[]  NTsProdOutMin=[]  NTsProdOutMax=[]  UintegralTsProdOutMin=[]  UintegralTsProdOutMax=[]  UngainTsProdOutMin=[]  UngainTsProdOutMax=[]  ClampingZeroOutDataTypeStr=Inherit: Inherit via back propagation  ClampingZeroOutMin=[]  ClampingZeroOutMax=[]  FilterDenConstantOutDataTypeStr=Inherit: Inherit via back propagation  FilterDenConstantOutMin=[]  FilterDenConstantOutMax=[]  PCopyOutDataTypeStr=Inherit: Inherit via back propagation  PCopyOutMin=[]  PCopyOutMax=[]  NCopyOutDataTypeStr=Inherit: Inherit via back propagation  NCopyOutMin=[]  NCopyOutMax=[]  IntegratorContinuousStateAttributes=''  IntegratorStateMustResolveToSignalObject=off  IntegratorRTWStateStorageClass=Auto  FilterContinuousStateAttributes=''  FilterStateMustResolveToSignalObject=off  FilterRTWStateStorageClass=Auto  ParallelPVariant=InternalParameters  IdealPVariant=Disabled  IVariant=InternalParameters  DVariant=InternalParameters  IntegratorVariant=Discrete  SatVariant=Enabled  AWVariant=DiscClampingParallel  PCopyVariant=Disabled  TRVariant=Disabled  FdbkBlocksVariant=Forward  IdealPFdbkVariant=Disabled  SatFdbkVariant=Disabled  DerivativeFilterVariant=ForwardEulerFilter  NVariant=InternalParameters  NCopyVariant=Disabled  FilterICVariant=InternalICsFilter  IntegratorICVariant=InternalICs  ExternalResetVariant=Disabled  TRSumVariant=Passthrough  SumFdbkVariant=Disabled  SumVariant=Sum_PID  TsampFilterVariant=InternalTs  TsampNgainVariant=Passthrough  TsampIntegralVariant=Disabled_SignalSpec  ExternalSaturationOutDataTypeStr=Inherit: Same as second input
      settings: AttributesFormatString=P: %<P>, I: %<I>, D:%<D>
  Accel Cmd : Outport
  wires:
  Add1/1 -> Demux1/1  "Velocity Error"
  PID_Vz/1 -> Mux/3
  Demux1/1 -> PID_Vx/1
  PID_Vy/1 -> Mux/2
  Velocity Cmd/1 -> Add1/1
  Demux1/3 -> PID_Vz/1
  Mux/1 -> Accel Cmd/1
  PID_Vx/1 -> Mux/1
  Demux1/2 -> PID_Vy/1
  Bus Selector1/1 -> Add1/2  "<WorldVelocity>"
  QuadRotorState/1 -> Bus Selector1/1

== stateflow chart uavSafeLanding/Safe Landing ==
  state EmergencyMode
    state FollowMode [parallel]
      settings: executionOrder=1
    state InitPos [parallel]
      en:
      poseInit = poseYPR;
      settings: executionOrder=3
    state MapMode [parallel]
      settings: executionOrder=2
    (default) -> FollowMode
  state HoverAndDetect
    state HoverMode [parallel]
      en:
      position = pose(1:3);
      scans = 0;
      du:
      LAP = position;
      settings: executionOrder=1
    state LandDetection [parallel]
      en,du:
      curPosnNED = position(1:3);
      initPosnNED = poseInit(1:3);
      curPosnENU = [curPosnNED(2); curPosnNED(1); ...
      -curPosnNED(3)];
      initPosnENU = [initPosnNED(2); initPosnNED(1); ...
      -initPosnNED(3)];
      positionDiff = curPosnENU - initPosnENU;
      [isDetected,LandingPos,isSuitable] = ...
      safeLand(pcMap, positionDiff);
      LandingPos = pcToWorld(LandingPos,...
      poseInit);
      settings: executionOrder=2
  state LandMode
    en,du:
    LAP = [LandingPos(1:2) height]';
    uavDistXY = dist(LAP(1:2),pose(1:2));
  state MissionMode
  state LandZone
    LAP = [LandingPos(1:2) 0]';
    stopSim(LAP(3), pose(3));
  state stopSim(LAP, pose) [function]
  state [isDetected,landPos,isSuitable] = safeLand(a,b) [function]
  (default) -> MissionMode
  HoverAndDetect -> LandMode [order 1] : [%after(20,sec)
      | isDetected]
      | {height = pose(3);}
  EmergencyMode -> HoverAndDetect : [isMapDone]
  LandMode -> LandZone : [uavDistXY < 1]
  MissionMode -> EmergencyMode : [mode == 2]
  HoverAndDetect -> EmergencyMode [order 2] : [~isDetected]
  data: sf_internal_action_state_placeholder_data local double size=1 =0; sf_internal_action_state_placeholder_data local double size=1 =0; sf_internal_action_state_placeholder_data local double size=1 =0; a function_input; b function_input; y function_output; LAP function_input double size=1; pose function_input double size=1; isDetected function_output; a function_input double size=[600000 3]; b function_input double size=[3 1]; landPos function_output; isSuitable function_output; bestLandLoc function_input; pos function_input; ptWorld function_output; LAP output double size=[3 1]; mission input; pose input; lookaheadDistance input; DesiredCourse output double size=[1 1]; DesiredYaw output double size=[1 1]; mode input; position local double size=[3 1]; scans local; LandingPos local; height local; uavDistXY local; ptCloud input size=[15 1800 3]; isMapDone output boolean size=[1 1]; pcMap output double size=[600000 3]; isSuitable output; isDetected local boolean size=[ 1 1]; poseYPR input; curPosnENU local; initPosnENU local; curPosnNED local; initPosnNED local; poseInit local; positionDiff local
  function y = dist(a, b):
    | function y = dist(a,b)
    |  
    | y = sqrt((a(1)-b(1))^2 + (a(2) - b(2))^2);
  function ptWorld = pcToWorld(bestLandLoc,pos):
    | function ptWorld = pcToWorld(bestLandLoc,pos)
    |  
    | 
    | initUAVOrientation = [pos(6) pos(5) pos(4)];
    | initUAVPosition = [pos(2) pos(1) pos(3)]; 
    | initUAVPose = rigidtform3d(initUAVOrientation, initUAVPosition);
    | ptWorld = pctransform(pointCloud(bestLandLoc),initUAVPose).Location;
    | 
    | ptWorld = [ptWorld(2) ptWorld(1) ptWorld(3)];

== matlab function uavSafeLanding/Controller/Attitude Control/Multirotor Acceleration Control ==
  data: acc input; roll output; pitch output; thrust output; yaw input; DroneMass parameter; Gravity parameter
function [roll, pitch, thrust] = accControl(acc, yaw, DroneMass, Gravity)

    xddot = acc(1);
    yddot = acc(2);
    zddot = acc(3);
    
    pitch = atan2((-xddot*cos(yaw)-yddot*sin(yaw)), ( -zddot + Gravity));
    roll = atan2(((-xddot*sin(yaw)+yddot*cos(yaw))*cos(pitch)), (-zddot+Gravity));
    
    roll_limit = 25*pi/180;
    pitch_limit = 25*pi/180;
    
    roll = min(roll_limit, max(-roll_limit, roll));
   
    pitch = min(pitch_limit, max(-pitch_limit, pitch));
    
    thrust = DroneMass*(-zddot+Gravity)/(cos(pitch)*cos(roll));
end
